simulink model "lvtest8"  (Simulink 7.1)
settings: Solver=ode45  StartTime=0.0  StopTime=50  RelTol=1e-2
values from neighbouring files (symbols this model uses):
  c1 = 1.5    [find_bigvalue.m]    (also in find_bigvalue1.m)
undefined symbols (not defined in the file or in its folder): c2, c3, c4, c5, c6, u0
libraries: wt_blockset_v3 x1, DRlib x1
settings Model: Creator=lv  LastModifiedBy=lv

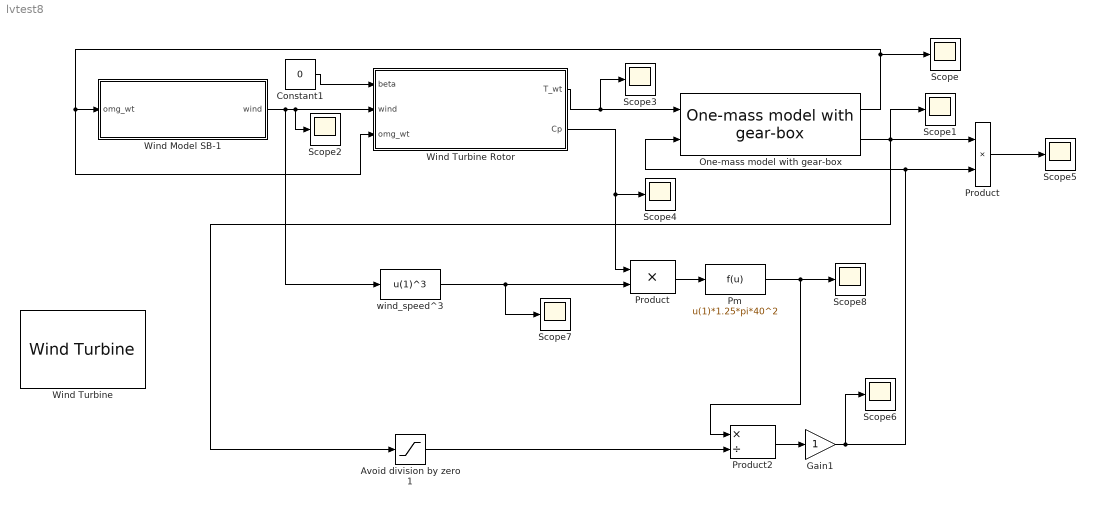
== system lvtest8 ==
  Avoid division by zero 1 : Saturate  UpperLimit=1e6  LowerLimit=1e-6  OutDataType=sfix(16)  OutScaling=2^0
  Constant1 : Constant  Value=0  OutDataType=sfix(16)  OutScaling=2^0
  Gain1 : Gain  ParameterDataType=sfix(16)  ParameterScaling=2^0  OutDataType=sfix(16)  OutScaling=2^0  SaturateOnIntegerOverflow=on  OutDataTypeStr=Inherit: Same as input  ParamDataTypeStr=Inherit: Same as input
  One-mass model with gear-box : wt_blockset_v3/Mechanical Components/One-mass model with gear-box  SystemSampleTime=-1  Jem=60  Jwt=12000  K=83.33  init_speed=1.87355
  Pm : Fcn  Expr=u(1)*1.25*pi*40^2
  Product : Product  OutDataType=sfix(16)  OutScaling=2^0  RndMeth=Zero
  "Product " : Product  OutDataType=sfix(16)  OutScaling=2^0  SaturateOnIntegerOverflow=on  OutDataTypeStr=Inherit: Same as first input
  Product2 : Product  Inputs=*/  OutDataType=sfix(16)  OutScaling=2^0  SaturateOnIntegerOverflow=on  OutDataTypeStr=Inherit: Same as first input
  Scope{,1..8} (9 alike) : Scope
      Scope settings: YMin=4.0189  YMax=4.0205
      Scope2 settings: YMin=13.4  YMax=15  SaveName=ScopeData2
      Scope3 settings: SaveName=ScopeData3
      Scope4 settings: SaveName=ScopeData4
      Scope5 settings: YMin=-595000  YMax=-530000  SaveName=ScopeData5
      Scope6 settings: SaveName=ScopeData6
      Scope7 settings: SaveName=ScopeData7
      Scope8 settings: SaveName=ScopeData8
  Wind Model SB-1 : Subsystem  AncestorBlock=wt_blockset_v3/Mechanical Components/Wind Model SB-1  TreatAsAtomicUnit=on  mask(Wind Model using Simulink Band-limited white noise generator){D_rotor=80, v_mean=13.5, roughness=600, turb_int=12, T_sample=0.05}
      mask prompts: D_rotor "Rotor diameter [m]"; v_mean "Average wind speed [m/sec]"; roughness "Length scale [m]"; turb_int "Turbulence intensity [%]"; T_sample "Sample time [sec]"
      mask help:
      | Implements a rotor wind model developped by RISOE National Laboratory based on Kaimal spectra. The model takes into account the rotational turbulences and the tower shadow.
      | This model uses the built-in band-limited white noise generator from Simulink with different seeds.
      mask init:
      | r = D_rotor/2;
      | sigma = v_mean*turb_int/100;
      | var = sigma^2;
      | c = roughness/(2*pi*v_mean);
      | d = r/v_mean;
      | trans=sigma*sqrt(roughness/v_mean);
      | random=[256, 894, 31];
      mask Display: disp('Wind\nModel\n(SB-1)')
  Wind Turbine : DRlib/Wind Generation/Wind Turbine  DialogController=POWERSYS.PowerSysDialog  SystemSampleTime=-1  Pnom=1.5e6  Pelec_base=1.5e6/0.9  wind_base=12  P_wind_base=0.73  speed_nom=1.2  pitch_angle=0  DisplayTurbChar=off  c1_c6="[0.51763          116          0.4            5           21     0.006795]"  cp_nom=0.48  lambda_nom=8.1
  Wind Turbine Rotor : Subsystem  AncestorBlock=wt_blockset_beta/Mechanical Components/Wind Turbine Rotor  mask(Aerodynamic model for wind turbine){R=40, ro_air=1.25, cut_in=3, cut_out=25, Tact=0}
      mask prompts: R "Blade radius [m]"; ro_air "Air density [kg m3]"; cut_in "Cut in speed [m/sec]"; cut_out "Cut out speed [m/sec]"; Tact "Time constant for pitch actuator [sec]"
      mask init:
      | %cq_table
      mask Display: plot(20,0,120,200,[45,35,35,45,75,75,45],[85,92,108,115,115,85,85],[55,50,70,65],[115,180,190,115],[55,50,70,65],[85,10,20,85],[75,85],[102,102],[75,85],[98,98],[105,85,85,105],[80,85,115,120])
  wind_speed^3 : Fcn  Expr=u(1)^3
  wires:
  Wind Model SB-1/1(wind) -> Wind Turbine Rotor/2(wind), Scope2/1, wind_speed^3/1
  Wind Turbine Rotor/1(T_wt) -> One-mass model with gear-box/1, Scope3/1
  One-mass model with gear-box/1 -> Scope/1, Wind Model SB-1/1(omg_wt), Wind Turbine Rotor/3(omg_wt)
  One-mass model with gear-box/2 -> Scope1/1, Product/1, Avoid division by zero 1/1
  Avoid division by zero 1/1 -> Product2/2
  wind_speed^3/1 -> Scope7/1, "Product "/2
  "Product "/1 -> Pm/1
  Pm/1 -> Product2/1, Scope8/1
  Product2/1 -> Gain1/1
  Gain1/1 -> Scope6/1, Product/2, One-mass model with gear-box/2
  Product/1 -> Scope5/1
  Wind Turbine Rotor/2(Cp) -> Scope4/1, "Product "/1
  Constant1/1 -> Wind Turbine Rotor/1(beta)

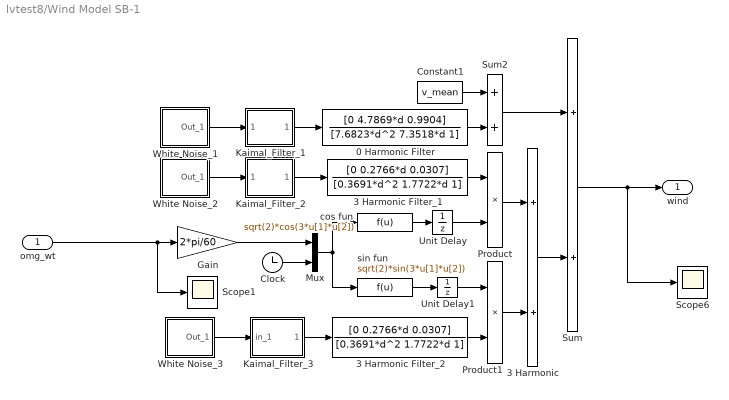
== system lvtest8/Wind Model SB-1 ==
  omg_wt : Inport  OutDataType=sfix(16)  OutScaling=2^0
  0 Harmonic Filter : TransferFcn  Numerator=[0 4.7869*d 0.9904]  Denominator=[7.6823*d^2 7.3518*d 1]
  3 Harmonic : Sum  OutDataType=sfix(16)  OutScaling=2^0  SaturateOnIntegerOverflow=on  InputSameDT=on  OutDataTypeStr=Inherit: Same as first input
  3 Harmonic Filter_1 : TransferFcn  Numerator=[0 0.2766*d 0.0307]  Denominator=[0.3691*d^2 1.7722*d 1]
  3 Harmonic Filter_2 : TransferFcn  Numerator=[0 0.2766*d 0.0307]  Denominator=[0.3691*d^2 1.7722*d 1]
  Clock : Clock
  Constant1 : Constant  Value=v_mean  OutDataType=sfix(16)  OutScaling=2^0
  Gain : Gain  Gain=2*pi/60  ParameterDataType=sfix(16)  ParameterScaling=2^0  OutDataType=sfix(16)  OutScaling=2^0  SaturateOnIntegerOverflow=on  OutDataTypeStr=Inherit: Same as input  ParamDataTypeStr=Inherit: Same as input
  Kaimal_Filter_1 : Subsystem
  Kaimal_Filter_2 : Subsystem
  Kaimal_Filter_3 : Subsystem
  Mux : Mux  Inputs=2
  Product : Product  OutDataType=sfix(16)  OutScaling=2^0  SaturateOnIntegerOverflow=on  InputSameDT=on  OutDataTypeStr=Inherit: Same as first input
  Product1 : Product  OutDataType=sfix(16)  OutScaling=2^0  SaturateOnIntegerOverflow=on  InputSameDT=on  OutDataTypeStr=Inherit: Same as first input
  Scope1 : Scope
      settings: YMin=-2.25e+010  YMax=1.5e+010  SaveName=ScopeData22
  Scope6 : Scope
      settings: TimeRange=100  YMin=-9e+006  YMax=9e+006  SaveName=ScopeData39
  Sum : Sum  OutDataType=sfix(16)  OutScaling=2^0  SaturateOnIntegerOverflow=on  InputSameDT=on  OutDataTypeStr=Inherit: Same as first input
  Sum2 : Sum  OutDataType=sfix(16)  OutScaling=2^0  SaturateOnIntegerOverflow=on  InputSameDT=on  OutDataTypeStr=Inherit: Same as first input
  Unit Delay : UnitDelay  SampleTime=T_sample
  Unit Delay1 : UnitDelay  SampleTime=T_sample
  White Noise_1 : Subsystem  mask(Continuous White Noise.){Cov=[1], Ts=T_sample, seed=[random(1)]}
      mask prompts: Cov "Noise Power:"; Ts "Sample Time:"
      mask help:
      | White noise for continuous (s-domain) systems.
      | Band-limited using zero-order-hold.
      mask init:
      | r = rand(1,12); r2 = [r(1),r;r,r(12)]; t =[1:13;1:13];
      mask Help: Implemented using white noise into Zero-Order Hold block. The seed and power can be vectors of the same length to produce a vector of white noise sources. For faster simulation, set sample time to the highest value possible but in accordance with the fastest dynamics of system.
      mask Display: plot(t(:),r2(:))
  White Noise_2 : Subsystem  mask(Continuous White Noise.){@1=[1], @2=T_sample, @3=[random(2)]}
      mask prompts: @1 "Noise Power:"; @2 "Sample Time:"; @3 "Seed"
      mask help:
      | White noise for continuous (s-domain) systems.
      | Band-limited using zero-order-hold.
      mask init:
      | Cov = @1; Ts = @2; seed = @3; r = rand(1,12); r2 = [r(1),r;r,r(12)]; t =[1:13;1:13];
      mask Help: Implemented using white noise into Zero-Order Hold block. The seed and power can be vectors of the same length to produce a vector of white noise sources. For faster simulation, set sample time to the highest value possible but in accordance with the fastest dynamics of system.
      mask Display: plot(t(:),r2(:))
  White Noise_3 : Subsystem  mask(Continuous White Noise.){@1=[1], @2=T_sample, @3=[random(3)]}
      mask prompts: @1 "Noise Power:"; @2 "Sample Time:"; @3 "Seed"
      mask help:
      | White noise for continuous (s-domain) systems.
      | Band-limited using zero-order-hold.
      mask init:
      | Cov = @1; Ts = @2; seed = @3; r = rand(1,12); r2 = [r(1),r;r,r(12)]; t =[1:13;1:13];
      mask Help: Implemented using white noise into Zero-Order Hold block. The seed and power can be vectors of the same length to produce a vector of white noise sources. For faster simulation, set sample time to the highest value possible but in accordance with the fastest dynamics of system.
      mask Display: plot(t(:),r2(:))
  cos fun : Fcn  Expr=sqrt(2)*cos(3*u[1]*u[2])
  sin fun : Fcn  Expr=sqrt(2)*sin(3*u[1]*u[2])
  wind : Outport  OutDataType=sfix(16)  OutScaling=2^0  InitialOutput=[u0]
  wires:
  Kaimal_Filter_2/1(out_1) -> 3 Harmonic Filter_1/1
  Kaimal_Filter_3/1(out_1) -> 3 Harmonic Filter_2/1
  cos fun/1 -> Unit Delay/1
  sin fun/1 -> Unit Delay1/1
  Product/1 -> 3 Harmonic/1
  Product1/1 -> 3 Harmonic/2
  3 Harmonic Filter_2/1 -> Product1/2
  3 Harmonic/1 -> Sum/2
  0 Harmonic Filter/1 -> Sum2/2
  Sum2/1 -> Sum/1
  Constant1/1 -> Sum2/1
  Sum/1 -> Scope6/1, wind/1
  Kaimal_Filter_1/1(out_1) -> 0 Harmonic Filter/1
  White Noise_1/1(Out_1) -> Kaimal_Filter_1/1(in_1)
  White Noise_2/1(Out_1) -> Kaimal_Filter_2/1(in_1)
  White Noise_3/1(Out_1) -> Kaimal_Filter_3/1(in_1)
  3 Harmonic Filter_1/1 -> Product/1
  Mux/1 -> cos fun/1, sin fun/1
  omg_wt/1 -> Scope1/1, Gain/1
  Unit Delay/1 -> Product/2
  Unit Delay1/1 -> Product1/1
  Clock/1 -> Mux/2
  Gain/1 -> Mux/1

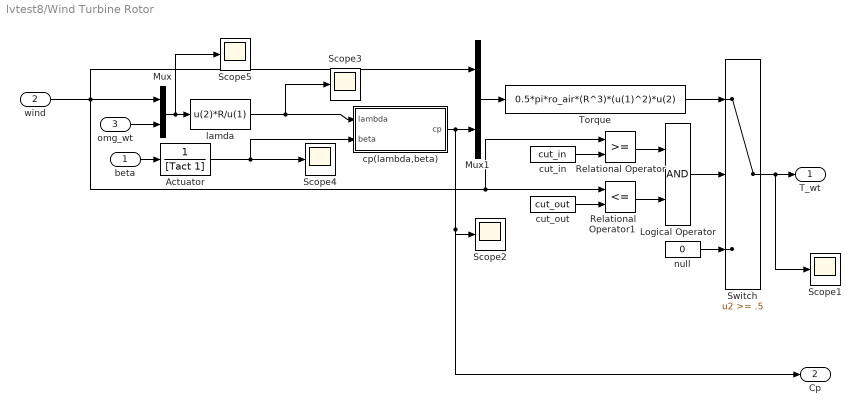
== system lvtest8/Wind Turbine Rotor ==
  beta : Inport  OutDataType=sfix(16)  OutScaling=2^0
  wind : Inport  Port=2  OutDataType=sfix(16)  OutScaling=2^0
  omg_wt : Inport  Port=3  OutDataType=sfix(16)  OutScaling=2^0
  Actuator : TransferFcn  Denominator=[Tact 1]
  Logical Operator : Logic
  Mux : Mux  Inputs=2
  Mux1 : Mux  Inputs=2
  Relational Operator : RelationalOperator  InputSameDT=on
  Relational Operator1 : RelationalOperator  Operator=<=  InputSameDT=on
  Scope{1..5} (5 alike) : Scope
      Scope1 settings: TimeRange=20  YMin=-1500000  YMax=1500000  SaveName=ScopeData19
      Scope2 settings: TimeRange=20  YMin=-1500000  YMax=1500000  SaveName=ScopeData11
      Scope3 settings: TimeRange=20  YMin=-1500000  YMax=1500000  SaveName=ScopeData12
      Scope4 settings: TimeRange=20  YMin=-1500000  YMax=1500000  SaveName=ScopeData14
      Scope5 settings: TimeRange=20  YMin=-1500000  YMax=1500000  SaveName=ScopeData9
  Switch : Switch  Threshold=.5  SaturateOnIntegerOverflow=on  InputSameDT=on
  Torque : Fcn  Expr=0.5*pi*ro_air*(R^3)*(u(1)^2)*u(2)
  cp(lambda,beta) : Subsystem
  cut_in : Constant  Value=cut_in  OutDataType=sfix(16)  OutScaling=2^0
  cut_out : Constant  Value=cut_out  OutDataType=sfix(16)  OutScaling=2^0
  lamda : Fcn  Expr=u(2)*R/u(1)
  null : Constant  Value=0  OutDataType=sfix(16)  OutScaling=2^0
  T_wt : Outport
  Cp : Outport  Port=2
  wires:
  beta/1 -> Actuator/1
  lamda/1 -> cp(lambda,beta)/1(lambda), Scope3/1
  wind/1 -> Mux1/1, Relational Operator1/1, Relational Operator/1, Mux/1
  Logical Operator/1 -> Switch/2
  null/1 -> Switch/3
  Torque/1 -> Switch/1
  Switch/1 -> Scope1/1, T_wt/1
  Relational Operator/1 -> Logical Operator/1
  Relational Operator1/1 -> Logical Operator/2
  cut_out/1 -> Relational Operator1/2
  cut_in/1 -> Relational Operator/2
  omg_wt/1 -> Mux/2
  Mux1/1 -> Torque/1
  Mux/1 -> lamda/1, Scope5/1
  cp(lambda,beta)/1(cp) -> Mux1/2, Scope2/1, Cp/1
  Actuator/1 -> cp(lambda,beta)/2(beta), Scope4/1

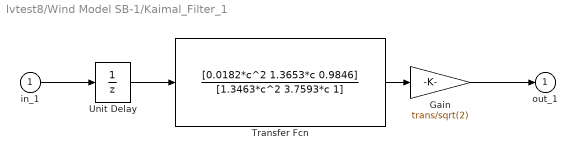
== system lvtest8/Wind Model SB-1/Kaimal_Filter_1 ==
  in_1 : Inport  OutDataType=sfix(16)  OutScaling=2^0
  Gain : Gain  Gain=trans/sqrt(2)  ParameterDataType=sfix(16)  ParameterScaling=2^0  OutDataType=sfix(16)  OutScaling=2^0  SaturateOnIntegerOverflow=on  OutDataTypeStr=Inherit: Same as input  ParamDataTypeStr=Inherit: Same as input
  Transfer Fcn : TransferFcn  Numerator=[0.0182*c^2 1.3653*c 0.9846]  Denominator=[1.3463*c^2 3.7593*c 1]
  Unit Delay : UnitDelay  SampleTime=T_sample
  out_1 : Outport  OutDataType=sfix(16)  OutScaling=2^0
  wires:
  Unit Delay/1 -> Transfer Fcn/1
  Gain/1 -> out_1/1
  in_1/1 -> Unit Delay/1
  Transfer Fcn/1 -> Gain/1

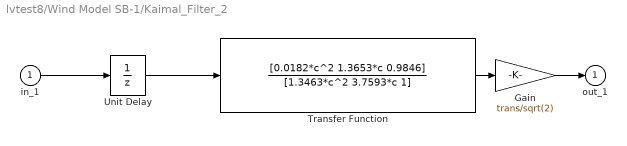
== system lvtest8/Wind Model SB-1/Kaimal_Filter_2 ==
  in_1 : Inport  OutDataType=sfix(16)  OutScaling=2^0
  Gain : Gain  Gain=trans/sqrt(2)  ParameterDataType=sfix(16)  ParameterScaling=2^0  OutDataType=sfix(16)  OutScaling=2^0  SaturateOnIntegerOverflow=on  OutDataTypeStr=Inherit: Same as input  ParamDataTypeStr=Inherit: Same as input
  Transfer Function : TransferFcn  Numerator=[0.0182*c^2 1.3653*c 0.9846]  Denominator=[1.3463*c^2 3.7593*c 1]
  Unit Delay : UnitDelay  SampleTime=T_sample
  out_1 : Outport  OutDataType=sfix(16)  OutScaling=2^0
  wires:
  Unit Delay/1 -> Transfer Function/1
  Gain/1 -> out_1/1
  in_1/1 -> Unit Delay/1
  Transfer Function/1 -> Gain/1

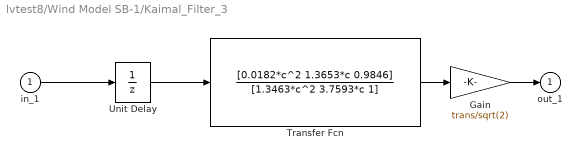
== system lvtest8/Wind Model SB-1/Kaimal_Filter_3 ==
  in_1 : Inport  OutDataType=sfix(16)  OutScaling=2^0
  Gain : Gain  Gain=trans/sqrt(2)  ParameterDataType=sfix(16)  ParameterScaling=2^0  OutDataType=sfix(16)  OutScaling=2^0  SaturateOnIntegerOverflow=on  OutDataTypeStr=Inherit: Same as input  ParamDataTypeStr=Inherit: Same as input
  Transfer Fcn : TransferFcn  Numerator=[0.0182*c^2 1.3653*c 0.9846]  Denominator=[1.3463*c^2 3.7593*c 1]
  Unit Delay : UnitDelay  SampleTime=T_sample
  out_1 : Outport  OutDataType=sfix(16)  OutScaling=2^0
  wires:
  Unit Delay/1 -> Transfer Fcn/1
  Gain/1 -> out_1/1
  in_1/1 -> Unit Delay/1
  Transfer Fcn/1 -> Gain/1

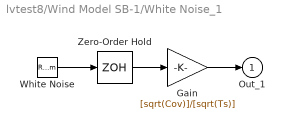
== system lvtest8/Wind Model SB-1/White Noise_1 ==
  Gain : Gain  Gain=[sqrt(Cov)]/[sqrt(Ts)]  ParameterDataType=sfix(16)  ParameterScaling=2^0  OutDataType=sfix(16)  OutScaling=2^0  SaturateOnIntegerOverflow=on  OutDataTypeStr=Inherit: Same as input  ParamDataTypeStr=Inherit: Same as input
  White Noise : RandomNumber  Seed=seed  SampleTime=Ts
  Zero-Order Hold : ZeroOrderHold  SampleTime=Ts
  Out_1 : Outport  OutDataType=sfix(16)  OutScaling=2^0
  wires:
  White Noise/1 -> Zero-Order Hold/1
  Gain/1 -> Out_1/1
  Zero-Order Hold/1 -> Gain/1

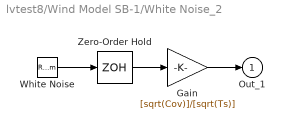
== system lvtest8/Wind Model SB-1/White Noise_2 ==
  Gain : Gain  Gain=[sqrt(Cov)]/[sqrt(Ts)]  ParameterDataType=sfix(16)  ParameterScaling=2^0  OutDataType=sfix(16)  OutScaling=2^0  SaturateOnIntegerOverflow=on  OutDataTypeStr=Inherit: Same as input  ParamDataTypeStr=Inherit: Same as input
  White Noise : RandomNumber  Seed=seed  SampleTime=Ts
  Zero-Order Hold : ZeroOrderHold  SampleTime=Ts
  Out_1 : Outport  OutDataType=sfix(16)  OutScaling=2^0
  wires:
  White Noise/1 -> Zero-Order Hold/1
  Gain/1 -> Out_1/1
  Zero-Order Hold/1 -> Gain/1

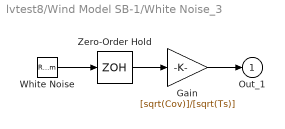
== system lvtest8/Wind Model SB-1/White Noise_3 ==
  Gain : Gain  Gain=[sqrt(Cov)]/[sqrt(Ts)]  ParameterDataType=sfix(16)  ParameterScaling=2^0  OutDataType=sfix(16)  OutScaling=2^0  SaturateOnIntegerOverflow=on  OutDataTypeStr=Inherit: Same as input  ParamDataTypeStr=Inherit: Same as input
  White Noise : RandomNumber  Seed=seed  SampleTime=Ts
  Zero-Order Hold : ZeroOrderHold  SampleTime=Ts
  Out_1 : Outport  OutDataType=sfix(16)  OutScaling=2^0
  wires:
  White Noise/1 -> Zero-Order Hold/1
  Gain/1 -> Out_1/1
  Zero-Order Hold/1 -> Gain/1

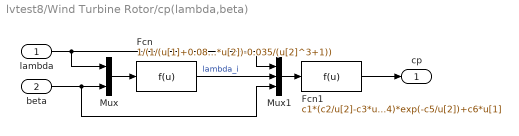
== system lvtest8/Wind Turbine Rotor/cp(lambda,beta) ==
  lambda : Inport  OutDataType=sfix(16)  OutScaling=2^0
  beta : Inport  Port=2  OutDataType=sfix(16)  OutScaling=2^0
  Fcn : Fcn  Expr=1/(1/(u[1]+0.08*u[2])-0.035/(u[2]^3+1))
  Fcn1 : Fcn  Expr=c1*(c2/u[2]-c3*u[3]-c4)*exp(-c5/u[2])+c6*u[1]
  Mux : Mux  Inputs=2
  Mux1 : Mux  Inputs=3
  cp : Outport  OutDataType=sfix(16)  OutScaling=2^0
  wires:
  Fcn/1 -> Mux1/2  "lambda_i"
  Fcn1/1 -> cp/1
  lambda/1 -> Mux1/1, Mux/1
  Mux1/1 -> Fcn1/1
  beta/1 -> Mux1/3, Mux/2
  Mux/1 -> Fcn/1
